simulink model "AdaptivePlantModel"  (R2020a)
settings: Solver=VariableStepAuto  StartTime=0.0  StopTime=10.0  RelTol=1e-3
values from neighbouring files (symbols this model uses):
  scenario = drivingScenario    [scenario_dritto.m]    (also in scenario_finale.m; scenario_sensors.m)
libraries: mpclib x1
settings Model: Creator=francesco  LastModifiedBy=francesco

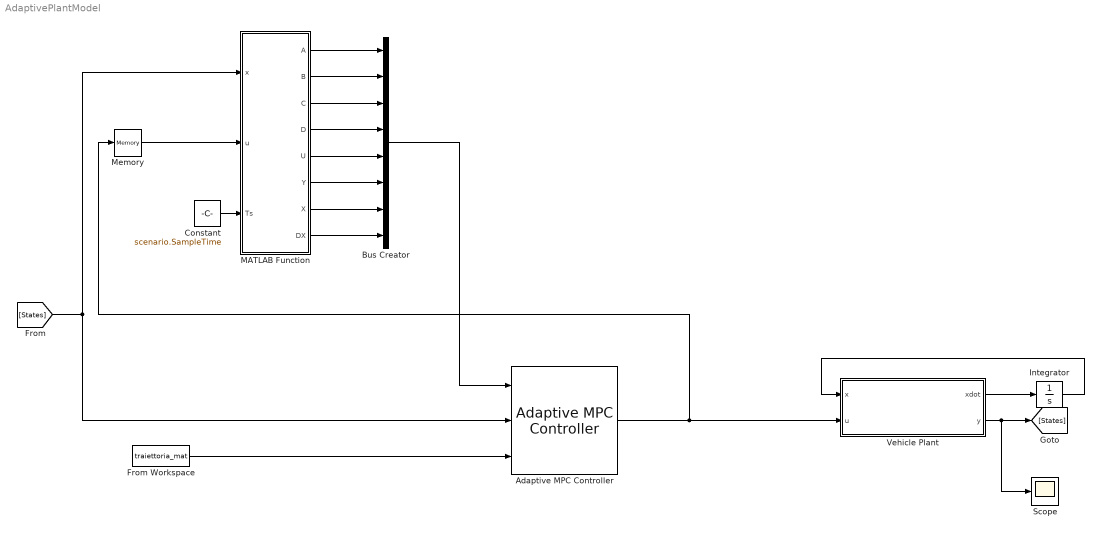
== system AdaptivePlantModel ==
  " Vehicle Plant" : MATLAB Function  TreatAsAtomicUnit=on
  Adaptive MPC Controller : mpclib/Adaptive MPC Controller  SCDEnableBlockLinearizationSpecification=on  mpcobj=mpc1  enable_value=0  updateMPCinCallerWorkspace=on  md_inport=off  mv_inport=off  uref_inport=off  return_cost=off  return_mvseq=off  return_qpstatus=off  return_xseq=off  return_state=off  return_ovseq=off  state_inport=off  isltv_plant=off  umin_inport=off  umax_inport=off  ymin_inport=off  ymax_inport=off  cc_inport=off  ywt_inport=off  uwt_inport=off  duwt_inport=off  rhoeps_inport=off  pm_inport=off  MaximumP=10  HorizonChoice=FixedHorizon  BlockDataType=double  SampleTimeInherited=off  switch_inport=off
  Bus Creator : BusCreator  Inputs=8
  Constant : Constant  Value=scenario.SampleTime
  From Workspace : FromWorkspace  VariableName=traiettoria_mat
  Integrator : Integrator
  MATLAB Function : MATLAB Function  TreatAsAtomicUnit=on
  Memory : Memory
  Scope : Scope
  wires:
  From Workspace/1 -> Adaptive MPC Controller/3
  " Vehicle Plant"/2(y) -> Scope/1, [States]
  [States] -> MATLAB Function/1(x), Adaptive MPC Controller/2
  Constant/1 -> MATLAB Function/3(Ts)
  Memory/1 -> MATLAB Function/2(u)
  Adaptive MPC Controller/1 -> Memory/1, " Vehicle Plant"/2(u)
  " Vehicle Plant"/1(xdot) -> Integrator/1
  Integrator/1 -> " Vehicle Plant"/1(x)
  Bus Creator/1 -> Adaptive MPC Controller/1
  MATLAB Function/1(A) -> Bus Creator/1
  MATLAB Function/2(B) -> Bus Creator/2
  MATLAB Function/3(C) -> Bus Creator/3
  MATLAB Function/4(D) -> Bus Creator/4
  MATLAB Function/5(U) -> Bus Creator/5
  MATLAB Function/6(Y) -> Bus Creator/6
  MATLAB Function/7(X) -> Bus Creator/7
  MATLAB Function/8(DX) -> Bus Creator/8

== matlab function AdaptivePlantModel/MATLAB Function ==
  data: x input; u input; A output; Ts input; B output; C output; D output; U output; Y output; X output; DX output
function [A,B,C,D,U,Y,X,DX] = fcn(x,u,Ts)
[Ac,Bc,Cd,Dd,U,Y,X,DX] = obstacleVehicleModelDT(Ts,x,u);

== matlab function AdaptivePlantModel/ Vehicle Plant ==
  data: x input; xdot output; u input; y output
function [xdot,y] = obstacleVehicleModelCT(x,u)
% The ego car has rectangular shaper with a length of 5 meters and width of
% 2 meters. The model has four states:
%
% * |xPos| - Global horizontal position of the car center
% * |yPos| - Global vertical position of the car center
% * |theta| - Heading angle of the car (0 when facing east, counterclockwise positive)
% * |V| - Speed of the car (positve)
%
% There are two manipulated variables:
%
% * |throttle| - Throttle (positive when accelerating, negative when braking)
% * |delta| - Steering angle change (counterclockwise positive)
%

%#codegen
carLength = egoVehicle.Length;
theta = x(3);
V = x(4);
delta = u(2);
A = [ 0, 0, -V*sin(theta), cos(theta);
      0, 0,  V*cos(theta), sin(theta);
      0, 0, 0,             tan(delta)/carLength;
      0, 0, 0,             0];
B = [0  , 0;
     0  , 0;
     0  , (V*(tan(delta)^2 + 1))/carLength;
     0.5, 0];
C = eye(4);
D = zeros(4,2);
xdot = A*x + B*u;
y = C*x + D*u;
